simulink model "pendulumNLMPC"  (R2022b)
settings: Solver=ode45  StartTime=0.0  StopTime=10  RelTol=1e-3
values from neighbouring files (symbols this model uses):
  x0 = [1.5;1]    [pendulumControl.m]
libraries: mpclib x1, slident x1
settings Model: Creator=rchen  LastModifiedBy=etzorako

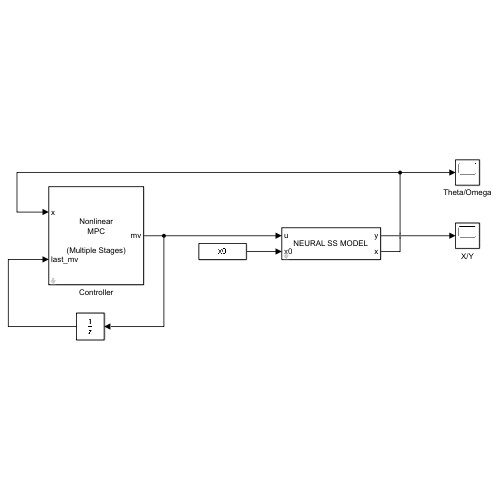
[thumbnail: Simulink's stored preview of the top-level diagram]
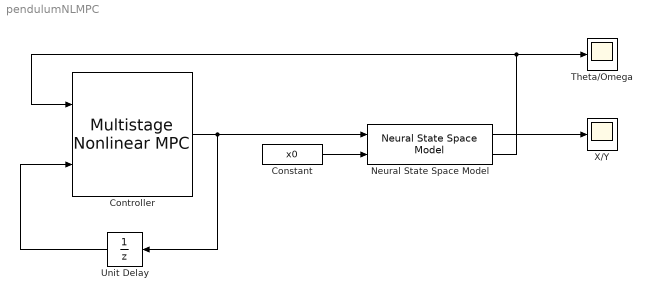
== system pendulumNLMPC ==
  Constant : Constant  Value=x0
  Controller : mpclib/Multistage Nonlinear MPC  nlmpcobj=nlmpcobj  UseObjectTs=on  UseMEX=off  md_enabled=off  stateparam_enabled=off  stageparam_enabled=off  cost_enabled=off  mvseq_enabled=off  stateseq_enabled=off  slack_enabled=off  status_enabled=off  mv_min=off  mv_max=off  mvrate_min=off  mvrate_max=off  state_min=off  state_max=off  terminal_state=off  nlp_initialize=off
  Neural State Space Model : slident/Models/Neural State Space Model  sys=obj  x0type=external  ic=0  returnx=on  returndx=off  domain=CT
  Theta/Omega : Scope
  Unit Delay : UnitDelay  SampleTime=-1  HasFrameUpgradeWarning=on
  X/Y : Scope
  wires:
  Controller/1 -> Neural State Space Model/1, Unit Delay/1
  Unit Delay/1 -> Controller/2
  Neural State Space Model/2 -> Theta/Omega/1, Controller/1
  Neural State Space Model/1 -> X/Y/1
  Constant/1 -> Neural State Space Model/2
